simulink model "sub_1"  (Simulink 9.2)
settings: Solver=ode45  StartTime=0.0  StopTime=0.022  RelTol=1e-3  EnableMultiTasking=on
settings Model: Creator=student  LastModifiedBy=murad
settings OptimizationCC: ExpressionDepthLimit=2147483647
settings DebuggingCC: SolverPrmCheckMsg=warning

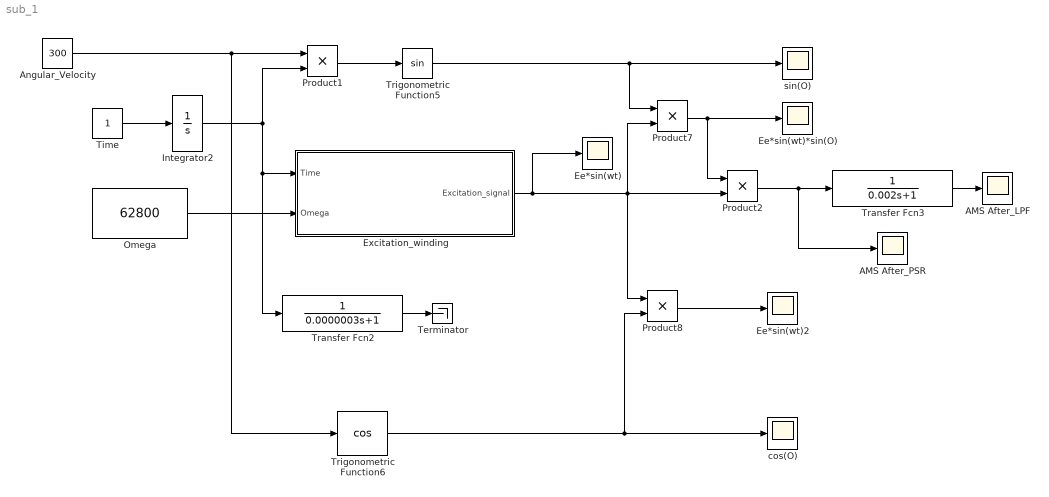
== system sub_1 ==
  AMS After_LPF : Scope
  AMS After_PSR : Scope
  Angular_Velocity : Constant  Value=300
  Ee*sin(wt) : Scope
  Ee*sin(wt)*sin(O) : Scope
  Ee*sin(wt)2 : Scope
  Excitation_winding : Subsystem
  Integrator2 : Integrator
  Omega : Constant  Value=62800
  Product{1..2,7..8} (4 alike) : Product  RndMeth=Zero
  Terminator : Terminator
  Time : Constant
  Transfer Fcn2 : TransferFcn  Denominator=[0.0000003 1]
  Transfer Fcn3 : TransferFcn  Denominator=[0.002 1]
  Trigonometric Function5 : Trigonometry
  Trigonometric Function6 : Trigonometry  Operator=cos
  cos(O) : Scope
  sin(O) : Scope
  wires:
  Product7/1 -> Product2/1, Ee*sin(wt)*sin(O)/1
  Trigonometric Function5/1 -> sin(O)/1, Product7/1
  Integrator2/1 -> Product1/2, Transfer Fcn2/1, Excitation_winding/1(Time)
  Omega/1 -> Excitation_winding/2(Omega)
  Trigonometric Function6/1 -> cos(O)/1, Product8/2
  Excitation_winding/1(Excitation_signal) -> Ee*sin(wt)/1, Product2/2, Product7/2, Product8/1
  Time/1 -> Integrator2/1
  Product1/1 -> Trigonometric Function5/1
  Angular_Velocity/1 -> Trigonometric Function6/1, Product1/1
  Transfer Fcn2/1 -> Terminator/1
  Product8/1 -> Ee*sin(wt)2/1
  Product2/1 -> AMS After_PSR/1, Transfer Fcn3/1
  Transfer Fcn3/1 -> AMS After_LPF/1

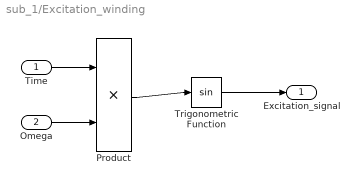
== system sub_1/Excitation_winding ==
  Time : Inport
  Omega : Inport  Port=2
  Product : Product  RndMeth=Zero
  Trigonometric Function : Trigonometry
  Excitation_signal : Outport
  wires:
  Omega/1 -> Product/2
  Trigonometric Function/1 -> Excitation_signal/1
  Time/1 -> Product/1
  Product/1 -> Trigonometric Function/1
